simulink model "AeroCoeffsNew"  (R2020b)
settings: Solver=VariableStepAuto  StartTime=0.0  StopTime=50  FixedStep=0.1  RelTol=1e-3
values from neighbouring files (symbols this model uses):
  A_2 = [0  0  0; 0  0  0; 0  0  0]    [Angular_gust.mat]    (also in Linear_gust.mat; Real_Values.m = zeros(3); Trial_Script.m = zeros(3); TryingNewAeroCoeffs.m = zeros(3))
  A_kal = [0 0 0 0 0 0 0 0 0 0 0 0 ... (36 elements, 6x6)]    [Angular_gust.mat]    (also in Linear_gust.mat; Real_Values.m = [0 0 0 1 0 0; Trial_Script.m = [0 0 0 1 0 0; TryingNewAeroCoeffs.m = [0 0 0 1 0 0)
  B_2 = [0.0024294842205  2.57653534931e-06  6.44659625064e-05; 0  -0.000916808772026  -2.10833406567e-07; 0  0  -0.000799328564006]    [Angular_gust.mat]    (also in Linear_gust.mat; Real_Values.m = I_inv; Trial_Script.m = I_inv; TryingNewAeroCoeffs.m = I_inv)
  B_kal = [0 0 0 0 0 0 0 0 0 0 0 0 ... (36 elements, 6x6)]    [Angular_gust.mat]    (also in Linear_gust.mat; Real_Values.m = [0 0 0 0 0 0; Trial_Script.m = [0 0 0 0 0 0; TryingNewAeroCoeffs.m = [0 0 0 0 0 0)
  C_2 = [1  0  0; 0  1  0; 0  0  1]    [Angular_gust.mat]    (also in Linear_gust.mat; Real_Values.m = eye(3); Trial_Script.m = eye(3); TryingNewAeroCoeffs.m = eye(3))
  C_kal = [1 0 0 0 0 0 0 1 0 0 0 0 ... (36 elements, 6x6)]    [Angular_gust.mat]    (also in Linear_gust.mat; Real_Values.m = eye(6); Trial_Script.m = eye(6); TryingNewAeroCoeffs.m = eye(6))
  D_2 = [0  0  0; 0  0  0; 0  0  0]    [Angular_gust.mat]    (also in Linear_gust.mat; Real_Values.m = zeros(3); Trial_Script.m = zeros(3); TryingNewAeroCoeffs.m = zeros(3))
  D_kal = [0 0 0 0 0 0 0 0 0 0 0 0 ... (36 elements, 6x6)]    [Angular_gust.mat]    (also in Linear_gust.mat; Real_Values.m = zeros(6); Trial_Script.m = zeros(6); TryingNewAeroCoeffs.m = zeros(6))
  delta_time = 0.0178961433409    [Angular_gust.mat]    (also in Linear_gust.mat; Real_Values.m = time/length(xdata); Trial_Script.m = time/length(xdata); TryingNewAeroCoeffs.m = time/length(xdata))
  Fb1_l = -2600    [Angular_gust.mat]    (also in Linear_gust.mat; Real_Values.m = -260; Trial_Script.m; TryingNewAeroCoeffs.m)
  Fb1_u = 2600    [Angular_gust.mat]    (also in Linear_gust.mat; Real_Values.m = 260; Trial_Script.m; TryingNewAeroCoeffs.m)
  Fb2_l = -2600    [Angular_gust.mat]    (also in Linear_gust.mat; Real_Values.m = -260; Trial_Script.m; TryingNewAeroCoeffs.m)
  Fb2_u = 2600    [Angular_gust.mat]    (also in Linear_gust.mat; Real_Values.m = 260; Trial_Script.m; TryingNewAeroCoeffs.m)
  Fb3_l = -3200    [Angular_gust.mat]    (also in Linear_gust.mat; Real_Values.m = -320; Trial_Script.m; TryingNewAeroCoeffs.m)
  Fb3_u = 3200    [Angular_gust.mat]    (also in Linear_gust.mat; Real_Values.m = 320; Trial_Script.m; TryingNewAeroCoeffs.m)
  Fb4_l = -3200    [Angular_gust.mat]    (also in Linear_gust.mat; Real_Values.m = -320; Trial_Script.m; TryingNewAeroCoeffs.m)
  Fb4_u = 3200    [Angular_gust.mat]    (also in Linear_gust.mat; Real_Values.m = 320; Trial_Script.m; TryingNewAeroCoeffs.m)
  Fc1_l = -300    [Angular_gust.mat]    (also in Linear_gust.mat; Real_Values.m = -100; Trial_Script.m = -3000; TryingNewAeroCoeffs.m)
  Fc1_u = 300    [Angular_gust.mat]    (also in Linear_gust.mat; Real_Values.m = 100; Trial_Script.m = 3000; TryingNewAeroCoeffs.m)
  Fc2_l = -300    [Angular_gust.mat]    (also in Linear_gust.mat; Real_Values.m = -100; Trial_Script.m = -3000; TryingNewAeroCoeffs.m)
  Fc2_u = 300    [Angular_gust.mat]    (also in Linear_gust.mat; Real_Values.m = 100; Trial_Script.m = 3000; TryingNewAeroCoeffs.m)
  Fc3_l = -300    [Angular_gust.mat]    (also in Linear_gust.mat; Real_Values.m = -100; Trial_Script.m = -3000; TryingNewAeroCoeffs.m)
  Fc3_u = 300    [Angular_gust.mat]    (also in Linear_gust.mat; Real_Values.m = 100; Trial_Script.m = 3000; TryingNewAeroCoeffs.m)
  fprop = 1000    [Angular_gust.mat]    (also in Linear_gust.mat; TryingNewAeroCoeffs.m)
  Ft1_l = -5600    [Angular_gust.mat]    (also in Linear_gust.mat; Real_Values.m = -560; Trial_Script.m; TryingNewAeroCoeffs.m)
  Ft1_u = 5600    [Angular_gust.mat]    (also in Linear_gust.mat; Real_Values.m = 560; Trial_Script.m; TryingNewAeroCoeffs.m)
  Ft2_l = -5600    [Angular_gust.mat]    (also in Linear_gust.mat; Real_Values.m = -560; Trial_Script.m; TryingNewAeroCoeffs.m)
  Ft2_u = 5600    [Angular_gust.mat]    (also in Linear_gust.mat; Real_Values.m = 560; Trial_Script.m; TryingNewAeroCoeffs.m)
  Ft3_l = -3200    [Angular_gust.mat]    (also in Linear_gust.mat; Real_Values.m = -320; Trial_Script.m; TryingNewAeroCoeffs.m)
  Ft3_u = 3200    [Angular_gust.mat]    (also in Linear_gust.mat; Real_Values.m = 320; Trial_Script.m; TryingNewAeroCoeffs.m)
  Ft4_l = -3200    [Angular_gust.mat]    (also in Linear_gust.mat; Real_Values.m = -320; Trial_Script.m; TryingNewAeroCoeffs.m)
  Ft4_u = 3200    [Angular_gust.mat]    (also in Linear_gust.mat; Real_Values.m = 320; Trial_Script.m; TryingNewAeroCoeffs.m)
  g = 9.81    [Angular_gust.mat]    (also in Linear_gust.mat; Real_Values.m; Trial_Script.m; TryingNewAeroCoeffs.m)
  m = 941.102    [Angular_gust.mat]    (also in Linear_gust.mat; Real_Values.m; Trial_Script.m = 645; TryingNewAeroCoeffs.m)
  r_0 = [0 0 0]    [Angular_gust.mat]    (also in Linear_gust.mat; Real_Values.m = [0;0;0]; Trial_Script.m = [0;0;0]; TryingNewAeroCoeffs.m = [0;0;0])
  r_cgCatia = [0.0401998 0.00180957 -0.293434]    [Angular_gust.mat]    (also in Linear_gust.mat; Real_Values.m = TcgCatia*r_cgCatia; Trial_Script.m = [2; 0; 0]; TryingNewAeroCoeffs.m = TcgCatia*r_cgCatia)
  r_trajectory = [0 0 0]    [Angular_gust.mat]    (also in Linear_gust.mat; Real_Values.m = [0;0;0]; Trial_Script.m = [0;0;0]; TryingNewAeroCoeffs.m = [0;0;0])
  rho = 1.225    [Angular_gust.mat]    (also in Linear_gust.mat; Real_Values.m; Trial_Script.m; TryingNewAeroCoeffs.m)
  T = 10.5    [Angular_gust.mat]    (also in Linear_gust.mat; Real_Values.m; Trial_Script.m; TryingNewAeroCoeffs.m)
  t_finalgust = 17.9140394843    [Angular_gust.mat]    (also in Linear_gust.mat; Real_Values.m = time; TryingNewAeroCoeffs.m = time)
  TcgCatia = [1  0  0; 0  -1  0; 0  0  -1]    [Angular_gust.mat]    (also in Linear_gust.mat; Real_Values.m = [1 0 0; Trial_Script.m = [1 0 0; TryingNewAeroCoeffs.m = [1 0 0)
  time = 17.9140394843    [Angular_gust.mat]    (also in Linear_gust.mat; Real_Values.m = rdiff_abs/V0_shard; Trial_Script.m = abs(rdiff_shard(2)/V0_shard(2)); TryingNewAeroCoeffs.m = rdiff_abs/V0_shard)
  time_delay = 0.01    [Angular_gust.mat]    (also in Linear_gust.mat; Real_Values.m = 0.1; Trial_Script.m = 0.1; TryingNewAeroCoeffs.m)
  Tzy_Shard = [6.12323399574e-17  1  1.22464679915e-16; 1  -6.12323399574e-17  -7.49879891331e-33; 0  1.22464679915e-16  -1]    [Angular_gust.mat]    (also in Linear_gust.mat; Real_Values.m = [cos(pi/2) -sin(pi/2) 0; sin(pi/2) cos(pi/2) 0; 0 0 1]*[1 0 ; Trial_Script.m = [cos(pi/2) -sin(pi/2) 0; sin(pi/2) cos(pi/2) 0; 0 0 1]*[1 0 ; TryingNewAeroCoeffs.m = [cos(pi/2) -sin(pi/2) 0; sin(pi/2) cos(pi/2) 0; 0 0 1]*[1 0 )
  u0_final = 23.9559    [Angular_gust.mat]    (also in Linear_gust.mat; Real_Values.m = u_0(length(u_0)); TryingNewAeroCoeffs.m = u_0(length(u_0)))
  u1_final = -0.480858    [Angular_gust.mat]    (also in Linear_gust.mat; Real_Values.m = u_1(length(u_1)); TryingNewAeroCoeffs.m = u_1(length(u_1)))
  u2_final = -0.725589    [Angular_gust.mat]    (also in Linear_gust.mat; Real_Values.m = u_2(length(u_2)); TryingNewAeroCoeffs.m = u_2(length(u_2)))
  u_0 = [24.7775 24.7775 24.7775 24.7775 24.7775 24.7775 24.7775 24.7775 24.7775 24.7775 24.7775 24.7775 ... (1001 elements, 1001x1)]    [Angular_gust.mat]    (also in Linear_gust.mat; Real_Values.m = a(1:d_shard,1); Trial_Script.m = a(1:d_shard,1); TryingNewAeroCoeffs.m = a(1:d_shard,1))
  u_1 = [0.712897 0.712897 0.712897 0.712897 0.712897 0.712897 0.712897 0.712897 0.712897 0.712897 0.712897 0.712897 ... (1001 elements, 1001x1)]    [Angular_gust.mat]    (also in Linear_gust.mat; Real_Values.m = a(1:d_shard,2); Trial_Script.m = a(1:d_shard,2); TryingNewAeroCoeffs.m = a(1:d_shard,2))
  u_2 = [-0.504815 -0.504815 -0.504815 -0.504815 -0.504815 -0.504815 -0.504815 -0.504815 -0.504815 -0.504815 -0.504815 -0.504815 ... (1001 elements, 1001x1)]    [Angular_gust.mat]    (also in Linear_gust.mat; Real_Values.m = a(1:d_shard,3); Trial_Script.m = a(1:d_shard,3); TryingNewAeroCoeffs.m = a(1:d_shard,3))
  v_0 = [0 0 0]    [Angular_gust.mat]    (also in Linear_gust.mat; Real_Values.m = [0;0;0]; Trial_Script.m = [0;0;0]; TryingNewAeroCoeffs.m = [0;0;0])
  ZI_Cx = [4.10002314469 4.10486511138 4.10970707807 4.11454904475 4.11939101144 4.12423297813 4.12907494481 4.1339169115 4.13875887819 4.14360084487 4.14844281156 4.15328477825 ... (65341 elements, 361x181)]    [Angular_gust.mat]    (also in Linear_gust.mat; Real_Values.m = model_Cx(XI_Cx, YI_Cx); Trial_Script.m = model_Cx(XI_Cx, YI_Cx); TryingNewAeroCoeffs.m = model_Cx(XI_Cx, YI_Cx))
  ZI_Cy = [5.10662222372 5.15407485934 5.20152749496 5.24898013059 5.29643276621 5.34388540184 5.39133803746 5.43879067308 5.48624330871 5.53369594433 5.58114857996 5.62860121558 ... (65341 elements, 361x181)]    [Angular_gust.mat]    (also in Linear_gust.mat; Real_Values.m = model_Cy(XI_Cy, YI_Cy); Trial_Script.m = model_Cy(XI_Cy, YI_Cy); TryingNewAeroCoeffs.m = model_Cy(XI_Cy, YI_Cy))
  ZI_Cz = [-10.5947720774 -10.6317912004 -10.6688103235 -10.7058294465 -10.7428485695 -10.7798676926 -10.8168868156 -10.8539059387 -10.8909250617 -10.9279441847 -10.9649633078 -11.0019824308 ... (65341 elements, 361x181)]    [Angular_gust.mat]    (also in Linear_gust.mat; Real_Values.m = model_Cz(XI_Cz, YI_Cz); Trial_Script.m = model_Cz(XI_Cz, YI_Cz); TryingNewAeroCoeffs.m = model_Cz(XI_Cz, YI_Cz))
  ZI_p = [6.05111971338 6.06712776392 6.08313581446 6.099143865 6.11515191553 6.13115996607 6.14716801661 6.16317606715 6.17918411769 6.19519216823 6.21120021877 6.22720826931 ... (65341 elements, 361x181)]    [Angular_gust.mat]    (also in Linear_gust.mat; Real_Values.m = model_p(XI_p, YI_p); Trial_Script.m = model_p(XI_p, YI_p); TryingNewAeroCoeffs.m = model_p(XI_p, YI_p))
  ZI_q = [0.071083987219 0.054175962948 0.0372679386771 0.0203599144061 0.00345189013513 -0.0134561341358 -0.0303641584068 -0.0472721826778 -0.0641802069487 -0.0810882312197 -0.0979962554907 -0.114904279762 ... (65341 elements, 361x181)]    [Angular_gust.mat]    (also in Linear_gust.mat; Real_Values.m = model_q(XI_q, YI_q); Trial_Script.m = model_q(XI_q, YI_q); TryingNewAeroCoeffs.m = model_q(XI_q, YI_q))
  ZI_r = [-1.8762921931 -1.88364224017 -1.89099228723 -1.8983423343 -1.90569238136 -1.91304242842 -1.92039247549 -1.92774252255 -1.93509256961 -1.94244261668 -1.94979266374 -1.95714271081 ... (65341 elements, 361x181)]    [Angular_gust.mat]    (also in Linear_gust.mat; Real_Values.m = model_r(XI_r, YI_r); Trial_Script.m = model_r(XI_r, YI_r); TryingNewAeroCoeffs.m = model_r(XI_r, YI_r))
undefined symbols (not defined in the file or in its folder): Continuous, Time
libraries: dspsigops x11, simulink x9, fuzblock x3, pid_lib x3, sharedutil x1, mpclib x1, cstblocks x1, dspmathops x1, ctrlSharedLib x1
(part 1 of 2)
settings Model: Creator=Jonathan van Zyl  LastModifiedBy=Jonathan van Zyl

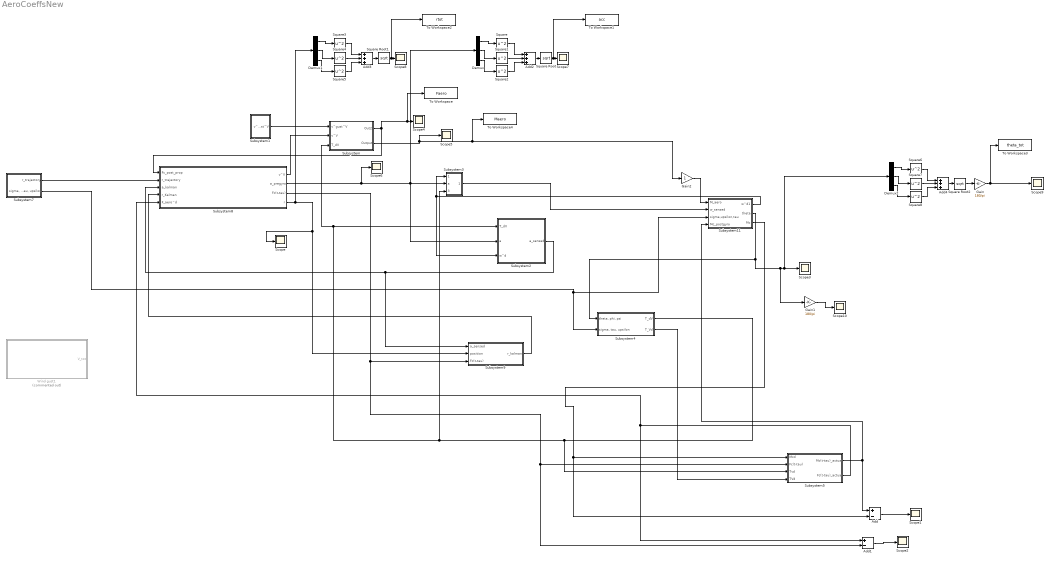
== system AeroCoeffsNew ==
  Add : Sum  Inputs=+-
  Add1 : Sum  Inputs=+-
  Add2 : Sum  Inputs=+++
  Add3 : Sum  Inputs=+++
  Add4 : Sum  Inputs=+++
  Demux : Demux  Outputs=3
  Demux1 : Demux  Outputs=3
  Demux2 : Demux  Outputs=3
  Gain : Gain  Gain=180/pi
  Gain1 : Gain  Gain=180/pi
  Gain2 : Gain
  Scope{,1..10} (11 alike) : Scope
  Square{,1..8} (9 alike) : Math  Operator=square  SaturateOnIntegerOverflow=on
  Square Root : Sqrt  SaturateOnIntegerOverflow=on
  Square Root1 : Sqrt  SaturateOnIntegerOverflow=on
  Square Root2 : Sqrt  SaturateOnIntegerOverflow=on
  Subsystem : Subsystem
  Subsystem1 : Subsystem
  Subsystem11 : Subsystem
  Subsystem2 : Subsystem
  Subsystem3 : Subsystem
  Subsystem4 : Subsystem
  Subsystem5 : Subsystem
  Subsystem7 : Subsystem
  Subsystem8 : Subsystem
  Subsystem9 : Subsystem
  To Workspace : ToWorkspace  VariableName=Faero  SaveFormat=Timeseries  SampleTime=-1
  To Workspace1 : ToWorkspace  VariableName=acc  SaveFormat=Timeseries  SampleTime=-1
  To Workspace2 : ToWorkspace  VariableName=rtot  SaveFormat=Timeseries  SampleTime=-1
  To Workspace3 : ToWorkspace  VariableName=theta_tot  SaveFormat=Timeseries  SampleTime=-1
  To Workspace4 : ToWorkspace  VariableName=Maero  SaveFormat=Timeseries  SampleTime=-1
  Wind gust1 : Subsystem  Commented=on
  wires:
  Subsystem2/1(a_sensed) -> Subsystem8/3(a_kalman), Subsystem9/1(a_sensed)
  Subsystem/2(Output) -> Scope5/1, Gain2/1, To Workspace4/1
  Subsystem/1(Out2) -> To Workspace/1, Scope4/1, Subsystem8/1(Fc_post_prop)
  Subsystem1/1(v^gust^V) -> Subsystem/1(v^gust^V)
  Subsystem4/1(T_dV) -> Subsystem5/3(Tvd), Subsystem/3(T_dV), Subsystem2/1(T_dV), Subsystem3/3(T_dV)
  Subsystem4/2(T_Vd) -> Subsystem5/4(TVd)
  Subsystem7/2("sigma, tau, upsilon") -> Subsystem11/3(sigma,upsilon,tau), Subsystem4/2("sigma, tau, upsilon")
  Subsystem8/3(Fc(t-tau)) -> Add1/2, Subsystem5/2(Fc(t-tau)), Subsystem9/3(Fc(t-tau))
  Subsystem7/1(r_trajectory) -> Subsystem8/2(r_trajectory)
  Subsystem5/2(Fc(t-tau)_actual) -> Add1/1, Subsystem8/5(F_aero^d)
  Subsystem8/1(v^V) -> Subsystem/2(v^V)
  Subsystem11/1(w^d1) -> Subsystem2/3(w^d), Subsystem3/1(w^d)
  Subsystem3/1(w^d1) -> Subsystem11/2(w_sensed)
  Subsystem5/1(Mc(t-tau)_actual) -> Subsystem11/4(Mc_postgyro), Add/1
  Subsystem11/3(Mc) -> Add/2, Subsystem5/1(Mcd)
  Subsystem9/1(r_kalman) -> Subsystem8/4(r_Kalman)
  Add/1 -> Scope1/1
  Add1/1 -> Scope2/1
  Demux/2 -> Square1/1
  Subsystem8/2(a_pregyro) -> Scope6/1, Demux/1, Subsystem3/2(a), Subsystem2/2(a)
  Demux/1 -> Square/1
  Demux/3 -> Square2/1
  Square Root/1 -> To Workspace1/1, Scope7/1
  Add2/1 -> Square Root/1
  Square2/1 -> Add2/3
  Square/1 -> Add2/1
  Square1/1 -> Add2/2
  Subsystem8/4(r) -> Demux1/1, Scope/1, Subsystem9/2(position)
  Demux1/2 -> Square4/1
  Demux1/1 -> Square3/1
  Add3/1 -> Square Root1/1
  Square4/1 -> Add3/2
  Square Root1/1 -> To Workspace2/1, Scope8/1
  Square3/1 -> Add3/1
  Demux1/3 -> Square5/1
  Square5/1 -> Add3/3
  Subsystem11/2(theta) -> Gain1/1, Demux2/1, Scope3/1, Subsystem4/1("theta, phi, psi")
  Demux2/2 -> Square7/1
  Demux2/1 -> Square6/1
  Add4/1 -> Square Root2/1
  Square7/1 -> Add4/2
  Gain/1 -> To Workspace3/1, Scope9/1
  Square6/1 -> Add4/1
  Demux2/3 -> Square8/1
  Square8/1 -> Add4/3
  Square Root2/1 -> Gain/1
  Gain1/1 -> Scope10/1
  Gain2/1 -> Subsystem11/1(M_aero)

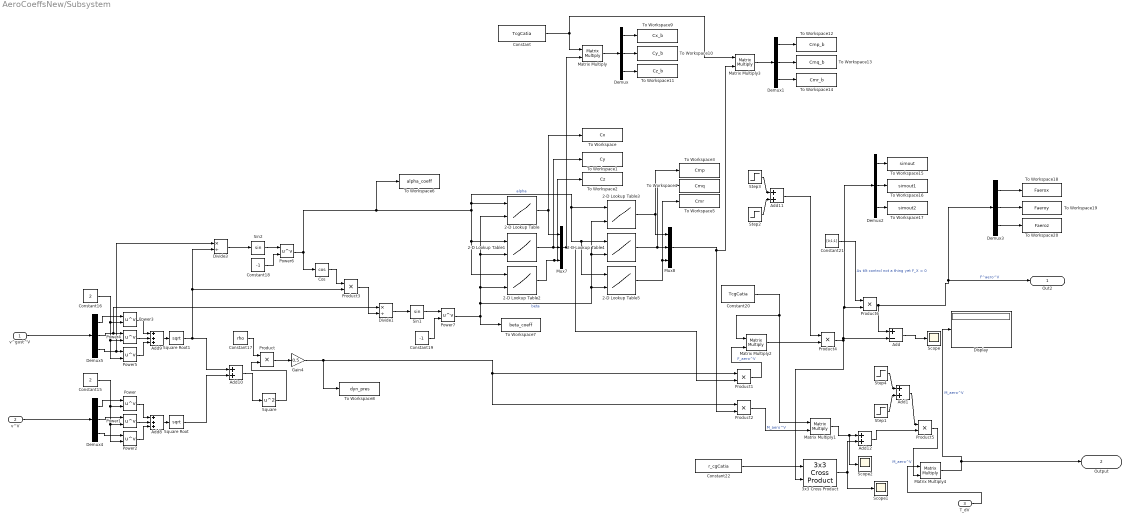
== system AeroCoeffsNew/Subsystem ==
  v^gust^V : Inport
  v^V : Inport  Port=2
  T_dV : Inport  Port=3
  2-D Lookup Table : Lookup_n-D  BreakpointsForDimension1=[-180:1:180]  BreakpointsForDimension2=[-90:1:90]  Table=ZI_Cx  InternalRulePriority=Speed  RndMeth=Simplest  InputSameDT=on
      settings: InputPortMap=u0,u1
  2-D Lookup Table1 : Lookup_n-D  BreakpointsForDimension1=[-180:1:180]  BreakpointsForDimension2=[-90:1:90]  Table=ZI_Cy  InternalRulePriority=Speed  RndMeth=Simplest  InputSameDT=on
      settings: InputPortMap=u0,u1
  2-D Lookup Table2 : Lookup_n-D  BreakpointsForDimension1=[-180:1:180]  BreakpointsForDimension2=[-90:1:90]  Table=ZI_Cz  InternalRulePriority=Speed  RndMeth=Simplest  InputSameDT=on
      settings: InputPortMap=u0,u1
  2-D Lookup Table3 : Lookup_n-D  BreakpointsForDimension1=[-180:1:180]  BreakpointsForDimension2=[-90:1:90]  Table=ZI_p  InternalRulePriority=Speed  RndMeth=Simplest  InputSameDT=on
      settings: InputPortMap=u0,u1
  2-D Lookup Table4 : Lookup_n-D  BreakpointsForDimension1=[-180:1:180]  BreakpointsForDimension2=[-90:1:90]  Table=ZI_q  InternalRulePriority=Speed  RndMeth=Simplest  InputSameDT=on
      settings: InputPortMap=u0,u1
  2-D Lookup Table5 : Lookup_n-D  BreakpointsForDimension1=[-180:1:180]  BreakpointsForDimension2=[-90:1:90]  Table=ZI_r  InternalRulePriority=Speed  RndMeth=Simplest  InputSameDT=on
      settings: InputPortMap=u0,u1
  3x3 Cross Product : sharedutil/3x3 Cross Product  aMode=aMode
      settings: SourceProductBaseCode=AE,PW,MT,UV,VE,VP
  Add : Sum  Inputs=+-
  Add{1,10..12} (4 alike) : Sum
  Add8 : Sum  Inputs=+++
  Add9 : Sum  Inputs=+++
  Constant : Constant  Value=TcgCatia
  Constant15 : Constant  Value=2
  Constant16 : Constant  Value=2
  Constant17 : Constant  Value=rho
  Constant18 : Constant  Value=-1
  Constant19 : Constant  Value=-1
  Constant20 : Constant  Value=TcgCatia
  Constant21 : Constant  Value=[0;1;1]
  Constant22 : Constant  Value=r_cgCatia
  Cos : Trigonometry  Operator=cos
  Demux{,1..5} (6 alike) : Demux  Outputs=3
  Display : Display
  Divide1 : Product  Inputs=*/
  Divide3 : Product  Inputs=*/
  Gain4 : Gain  Gain=0.5
  Matrix Multiply{,1..4} (5 alike) : Product  Multiplication=Matrix(*)
  Mux7 : Mux  Inputs=3
  Mux8 : Mux  Inputs=3
  Power{,1..7} (8 alike) : Math  Operator=pow  SaturateOnIntegerOverflow=on
  Product{,1..6} (7 alike) : Product
  Scope : Scope
  Scope1 : Scope
  Scope2 : Scope
  Sin1 : Trigonometry
  Sin2 : Trigonometry
  Square : Math  Operator=square  SaturateOnIntegerOverflow=on
  Square Root : Sqrt  SaturateOnIntegerOverflow=on
  Square Root1 : Sqrt  SaturateOnIntegerOverflow=on
  Step1 : Step  Time=0  SampleTime=0
  Step2 : Step  Time=0  SampleTime=0
  Step3 : Step  Time=time  After=-1  SampleTime=0
  Step4 : Step  Time=time  After=-1  SampleTime=0
  To Workspace : ToWorkspace  VariableName=Cx  SaveFormat=Timeseries  SampleTime=-1
  To Workspace1 : ToWorkspace  VariableName=Cy  SaveFormat=Timeseries  SampleTime=-1
  To Workspace10 : ToWorkspace  VariableName=Cy_b  SaveFormat=Timeseries  SampleTime=-1
  To Workspace11 : ToWorkspace  VariableName=Cz_b  SaveFormat=Timeseries  SampleTime=-1
  To Workspace12 : ToWorkspace  VariableName=Cmp_b  SaveFormat=Timeseries  SampleTime=-1
  To Workspace13 : ToWorkspace  VariableName=Cmq_b  SaveFormat=Timeseries  SampleTime=-1
  To Workspace14 : ToWorkspace  VariableName=Cmr_b  SaveFormat=Timeseries  SampleTime=-1
  To Workspace15 : ToWorkspace  VariableName=simout  SaveFormat=Timeseries  SampleTime=-1
  To Workspace16 : ToWorkspace  VariableName=simout1  SaveFormat=Timeseries  SampleTime=-1
  To Workspace17 : ToWorkspace  VariableName=simout2  SaveFormat=Timeseries  SampleTime=-1
  To Workspace18 : ToWorkspace  VariableName=Faerox  SaveFormat=Timeseries  SampleTime=-1
  To Workspace19 : ToWorkspace  VariableName=Faeroy  SaveFormat=Timeseries  SampleTime=-1
  To Workspace2 : ToWorkspace  VariableName=Cz  SaveFormat=Timeseries  SampleTime=-1
  To Workspace20 : ToWorkspace  VariableName=Faeroz  SaveFormat=Timeseries  SampleTime=-1
  To Workspace3 : ToWorkspace  VariableName=Cmp  SaveFormat=Timeseries  SampleTime=-1
  To Workspace4 : ToWorkspace  VariableName=Cmq  SaveFormat=Timeseries  SampleTime=-1
  To Workspace5 : ToWorkspace  VariableName=Cmr  SaveFormat=Timeseries  SampleTime=-1
  To Workspace6 : ToWorkspace  VariableName=alpha_coeff  SaveFormat=Timeseries  SampleTime=-1
  To Workspace7 : ToWorkspace  VariableName=beta_coeff  SaveFormat=Timeseries  SampleTime=-1
  To Workspace8 : ToWorkspace  VariableName=dyn_pres  SaveFormat=Timeseries  SampleTime=-1
  To Workspace9 : ToWorkspace  VariableName=Cx_b  SaveFormat=Timeseries  SampleTime=-1
  Out2 : Outport
  Output : Outport  Port=2
  wires:
  Demux5/1 -> Power3/1
  Constant21/1 -> Product6/1  "As tilt control not a thing yet F_X = 0"
  2-D Lookup Table3/1 -> To Workspace3/1, Mux8/1
  Constant17/1 -> Product/1
  Power5/1 -> Add9/3
  Product4/1 -> Demux2/1, Product6/2, Add/2, 3x3 Cross Product/2
  Power7/1 -> 2-D Lookup Table/2, 2-D Lookup Table1/2, 2-D Lookup Table2/2, 2-D Lookup Table3/2, 2-D Lookup Table4/2, 2-D Lookup Table5/2, To Workspace7/1  "beta"
  2-D Lookup Table2/1 -> To Workspace2/1, Mux7/3
  Power3/1 -> Add9/1
  Constant15/1 -> Power2/2, Power1/2, Power/2
  Sin1/1 -> Power7/1
  Square/1 -> Product/2
  Demux4/2 -> Power1/1
  Gain4/1 -> To Workspace8/1, Product2/1, Product1/1
  Square Root1/1 -> Product3/2, Divide3/2, Add10/1
  Product1/1 -> Matrix Multiply2/2  "F_aero^V"
  2-D Lookup Table1/1 -> To Workspace1/1, Mux7/2
  Add8/1 -> Square Root/1
  Cos/1 -> Product3/1
  3x3 Cross Product/1 -> Add12/2, Scope1/1
  Power2/1 -> Add8/3
  Add9/1 -> Square Root1/1
  Divide3/1 -> Sin2/1
  Mux7/1 -> Matrix Multiply/2, Product1/2
  Demux5/2 -> Divide1/1, Power4/1
  Product3/1 -> Divide1/2
  Constant22/1 -> 3x3 Cross Product/1
  Product2/1 -> Matrix Multiply1/2  "M_aero^V"
  Demux4/3 -> Power2/1
  Square Root/1 -> Add10/2
  Constant16/1 -> Power5/2, Power4/2, Power3/2
  2-D Lookup Table5/1 -> To Workspace5/1, Mux8/3
  v^gust^V/1 -> Demux5/1
  Divide1/1 -> Sin1/1
  Power1/1 -> Add8/2
  Constant20/1 -> Matrix Multiply1/1, Matrix Multiply2/1
  Power4/1 -> Add9/2
  Power/1 -> Add8/1
  2-D Lookup Table4/1 -> To Workspace4/1, Mux8/2
  Matrix Multiply1/1 -> Scope2/1, Add12/1
  Mux8/1 -> Matrix Multiply3/2, Product2/2
  Constant18/1 -> Power6/2
  Demux4/1 -> Power/1
  Product6/1 -> Add/1, Out2/1, Demux3/1  "F^aero^V"
  Demux5/3 -> Divide3/1, Power5/1
  Product/1 -> Gain4/1
  Power6/1 -> Cos/1, To Workspace6/1, 2-D Lookup Table/1, 2-D Lookup Table5/1, 2-D Lookup Table4/1, 2-D Lookup Table3/1, 2-D Lookup Table2/1, 2-D Lookup Table1/1  "alpha"
  Sin2/1 -> Power6/1
  Constant19/1 -> Power7/2
  2-D Lookup Table/1 -> Mux7/1, To Workspace/1
  Add10/1 -> Square/1
  Matrix Multiply4/1 -> Display/1, Output/1  "M_aero^V"
  T_dV/1 -> Matrix Multiply4/1
  v^V/1 -> Demux4/1
  Add/1 -> Scope/1
  Constant/1 -> Matrix Multiply3/1, Matrix Multiply/1
  Matrix Multiply/1 -> Demux/1
  Demux/1 -> To Workspace9/1
  Demux/2 -> To Workspace10/1
  Demux/3 -> To Workspace11/1
  Matrix Multiply3/1 -> Demux1/1
  Demux1/1 -> To Workspace12/1
  Demux1/2 -> To Workspace13/1
  Demux1/3 -> To Workspace14/1
  Demux2/1 -> To Workspace15/1
  Demux2/2 -> To Workspace16/1
  Demux2/3 -> To Workspace17/1
  Demux3/1 -> To Workspace18/1
  Demux3/2 -> To Workspace19/1
  Demux3/3 -> To Workspace20/1
  Step3/1 -> Add11/1
  Add11/1 -> Product4/1
  Step2/1 -> Add11/2
  Matrix Multiply2/1 -> Product4/2
  Add1/1 -> Product5/1
  Step1/1 -> Add1/2
  Step4/1 -> Add1/1
  Product5/1 -> Matrix Multiply4/2  "M_aero^V"
  Add12/1 -> Product5/2

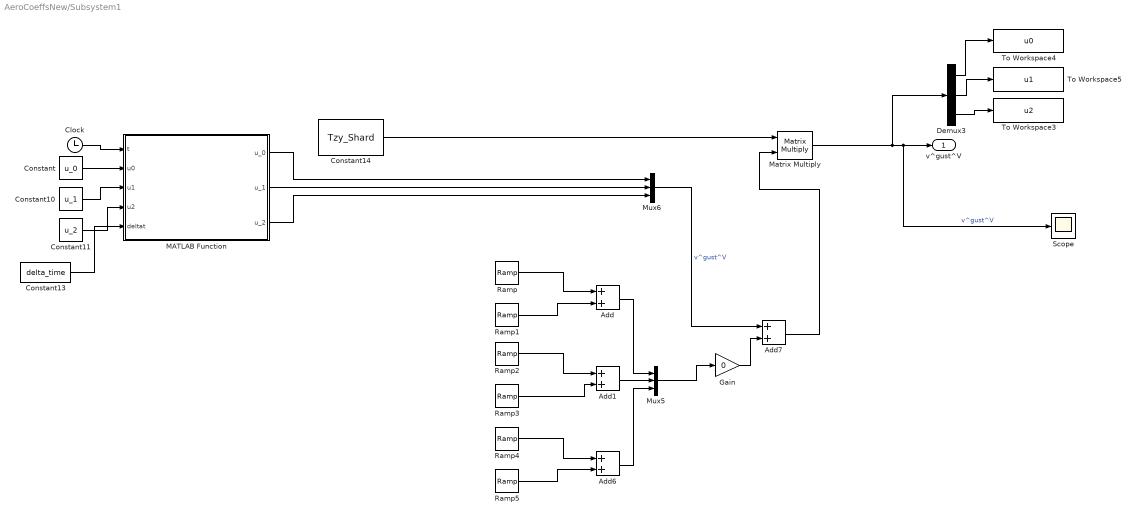
== system AeroCoeffsNew/Subsystem1 ==
  Add{,1,6..7} (4 alike) : Sum
  Clock : Clock
  Constant : Constant  Value=u_0
  Constant10 : Constant  Value=u_1
  Constant11 : Constant  Value=u_2
  Constant13 : Constant  Value=delta_time
  Constant14 : Constant  Value=Tzy_Shard
  Demux3 : Demux  Outputs=3
  Gain : Gain  Gain=0
  MATLAB Function : MATLAB Function  TreatAsAtomicUnit=on
  Matrix Multiply : Product  Multiplication=Matrix(*)
  Mux5 : Mux  Inputs=3
  Mux6 : Mux  Inputs=3
  Ramp : simulink/Sources/Ramp  slope=-1  start=t_finalgust  InitialOutput=0
  Ramp1 : simulink/Sources/Ramp  slope=1  start=t_finalgust + u0_final  InitialOutput=0
  Ramp2 : simulink/Sources/Ramp  slope=-1  start=t_finalgust  InitialOutput=0
  Ramp3 : simulink/Sources/Ramp  slope=1  start=t_finalgust + u1_final  InitialOutput=0
  Ramp4 : simulink/Sources/Ramp  slope=-1  start=t_finalgust  InitialOutput=0
  Ramp5 : simulink/Sources/Ramp  slope=1  start=t_finalgust + u2_final  InitialOutput=0
  Scope : Scope
  To Workspace3 : ToWorkspace  VariableName=u2  SaveFormat=Timeseries  SampleTime=-1
  To Workspace4 : ToWorkspace  VariableName=u0  SaveFormat=Timeseries  SampleTime=-1
  To Workspace5 : ToWorkspace  VariableName=u1  SaveFormat=Timeseries  SampleTime=-1
  v^gust^V : Outport
  wires:
  Add1/1 -> Mux5/2
  MATLAB Function/1(u_0) -> Mux6/1
  Add7/1 -> Matrix Multiply/2
  Constant13/1 -> MATLAB Function/5(deltat)
  Ramp4/1 -> Add6/1
  Ramp3/1 -> Add1/2
  Constant11/1 -> MATLAB Function/4(u2)
  Constant/1 -> MATLAB Function/2(u0)
  Ramp1/1 -> Add/2
  Mux5/1 -> Gain/1
  Constant14/1 -> Matrix Multiply/1
  MATLAB Function/2(u_1) -> Mux6/2
  Constant10/1 -> MATLAB Function/3(u1)
  Ramp/1 -> Add/1
  Matrix Multiply/1 -> Demux3/1, Scope/1, v^gust^V/1  "v^gust^V"
  Ramp5/1 -> Add6/2
  Add6/1 -> Mux5/3
  Clock/1 -> MATLAB Function/1(t)
  MATLAB Function/3(u_2) -> Mux6/3
  Add/1 -> Mux5/1
  Ramp2/1 -> Add1/1
  Mux6/1 -> Add7/1  "v^gust^V"
  Demux3/3 -> To Workspace3/1
  Demux3/2 -> To Workspace5/1
  Demux3/1 -> To Workspace4/1
  Gain/1 -> Add7/2

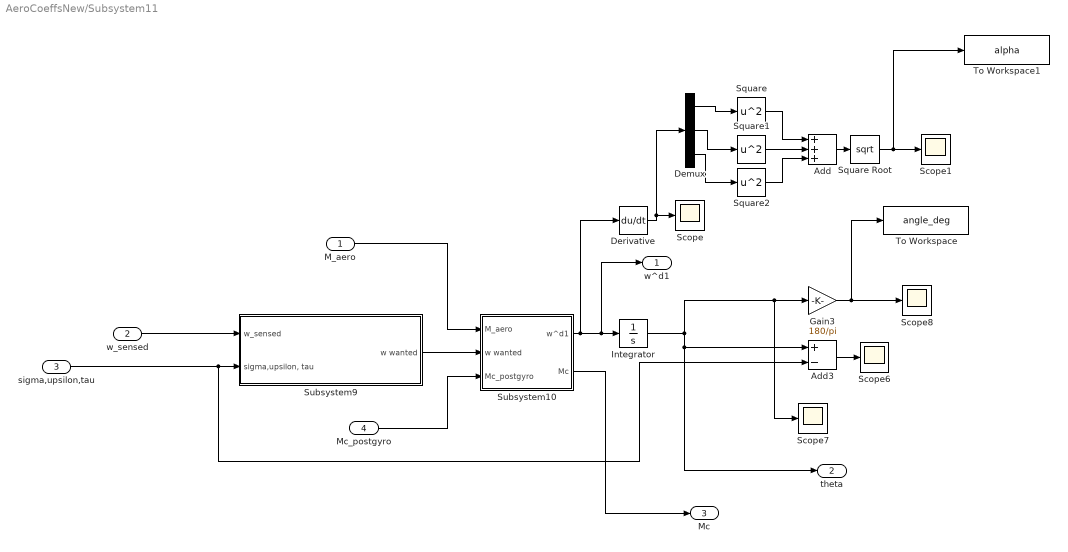
== system AeroCoeffsNew/Subsystem11 ==
  M_aero : Inport
  w_sensed : Inport  Port=2
  sigma,upsilon,tau : Inport  Port=3
  Mc_postgyro : Inport  Port=4
  Add : Sum  Inputs=+++
  Add3 : Sum  Inputs=+-
  Demux : Demux  Outputs=3
  Derivative : Derivative
  Gain3 : Gain  Gain=180/pi
  Integrator : Integrator
  Scope{,1,6..8} (5 alike) : Scope
  Square : Math  Operator=square  SaturateOnIntegerOverflow=on
  Square Root : Sqrt  SaturateOnIntegerOverflow=on
  Square1 : Math  Operator=square  SaturateOnIntegerOverflow=on
  Square2 : Math  Operator=square  SaturateOnIntegerOverflow=on
  Subsystem10 : Subsystem
  Subsystem9 : Subsystem
  To Workspace : ToWorkspace  VariableName=angle_deg  SaveFormat=Timeseries  SampleTime=-1
  To Workspace1 : ToWorkspace  VariableName=alpha  SaveFormat=Timeseries  SampleTime=-1
  w^d1 : Outport
  theta : Outport  Port=2
  Mc : Outport  Port=3
  wires:
  Gain3/1 -> To Workspace/1, Scope8/1
  M_aero/1 -> Subsystem10/1(M_aero)
  w_sensed/1 -> Subsystem9/1(w_sensed)
  Subsystem10/1(w^d1) -> Derivative/1, w^d1/1, Integrator/1
  sigma,upsilon,tau/1 -> Add3/2, Subsystem9/2("sigma,upsilon, tau")
  Integrator/1 -> theta/1, Add3/1, Gain3/1, Scope7/1
  Subsystem10/2(Mc) -> Mc/1
  Subsystem9/1(w wanted) -> Subsystem10/2(w wanted)
  Add3/1 -> Scope6/1
  Mc_postgyro/1 -> Subsystem10/3(Mc_postgyro)
  Derivative/1 -> Demux/1, Scope/1
  Demux/1 -> Square/1
  Demux/2 -> Square1/1
  Demux/3 -> Square2/1
  Square/1 -> Add/1
  Square1/1 -> Add/2
  Square2/1 -> Add/3
  Add/1 -> Square Root/1
  Square Root/1 -> To Workspace1/1, Scope1/1

== system AeroCoeffsNew/Subsystem2 ==
  T_dV : Inport
  a : Inport  Port=2
  w^d : Inport  Port=3
  Display1 : Display
  Display2 : Display
  MATLAB Function1 : MATLAB Function  Commented=on  TreatAsAtomicUnit=on
  Terminator5 : Terminator
  Terminator6 : Terminator
  Transpose1 : Math  Operator=transpose  SaturateOnIntegerOverflow=on
  Transpose2 : Math  Operator=transpose  SaturateOnIntegerOverflow=on
  Transpose3 : Math  Operator=transpose  SaturateOnIntegerOverflow=on
  a_sensed : Outport
  wires:
  a/1 -> Transpose1/1
  Transpose1/1 -> Display1/1, Transpose2/1, Display2/1  "a_sensed"
  Transpose3/1 -> Terminator5/1
  T_dV/1 -> Terminator6/1
  Transpose2/1 -> a_sensed/1  "a_sensed"
  w^d/1 -> Transpose3/1

== system AeroCoeffsNew/Subsystem3 ==
  w^d : Inport
  a : Inport  Port=2
  T_dV : Inport  Port=3
  Add : Sum  Inputs=+-
  Demux21 : Demux  Outputs=3
  Demux22 : Demux  Outputs=3
  MATLAB Function10 : MATLAB Function  TreatAsAtomicUnit=on
  Matrix Multiply4 : Product  Multiplication=Matrix(*)
  Mux14 : Mux  Inputs=3
  To Workspace : ToWorkspace  VariableName=gyro  SaveFormat=Timeseries  SampleTime=-1
  w^d1 : Outport
  wires:
  Demux21/3 -> MATLAB Function10/3(zvel)
  Demux22/1 -> MATLAB Function10/4(accx)
  Demux22/2 -> MATLAB Function10/5(accy)
  Demux22/3 -> MATLAB Function10/6(accz)
  MATLAB Function10/1(wx) -> Mux14/1
  Demux21/1 -> MATLAB Function10/1(xvel)
  MATLAB Function10/2(wy) -> Mux14/2
  Demux21/2 -> MATLAB Function10/2(yvel)
  MATLAB Function10/3(wz) -> Mux14/3
  Matrix Multiply4/1 -> Demux22/1
  Mux14/1 -> Add/2, w^d1/1  "w^d"
  T_dV/1 -> Matrix Multiply4/1
  a/1 -> Matrix Multiply4/2
  w^d/1 -> Add/1, Demux21/1
  Add/1 -> To Workspace/1

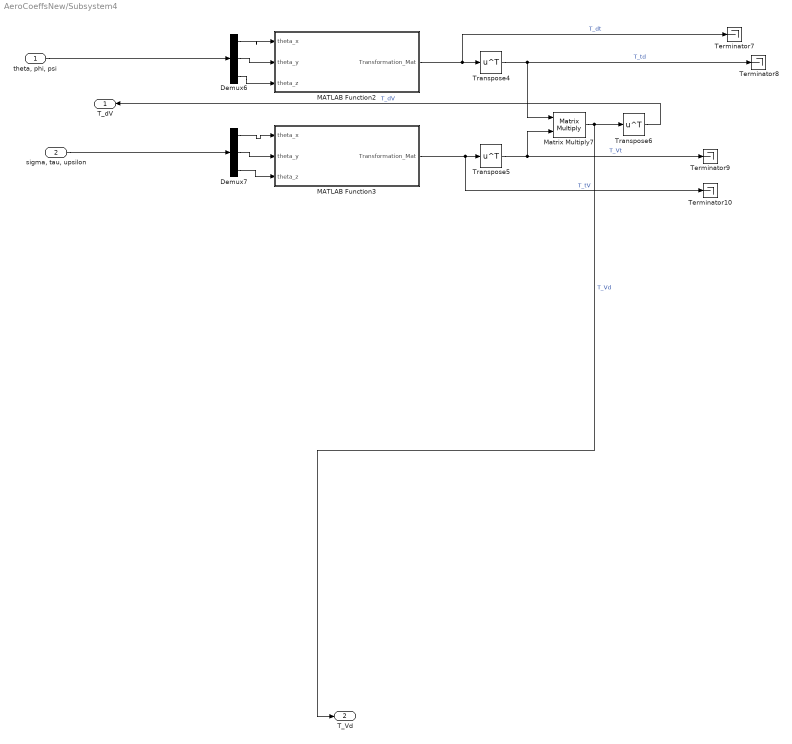
== system AeroCoeffsNew/Subsystem4 ==
  "theta, phi, psi" : Inport
  "sigma, tau, upsilon" : Inport  Port=2
  Demux6 : Demux  Outputs=3
  Demux7 : Demux  Outputs=3
  MATLAB Function2 : MATLAB Function  TreatAsAtomicUnit=on
  MATLAB Function3 : MATLAB Function  TreatAsAtomicUnit=on
  Matrix Multiply7 : Product  Multiplication=Matrix(*)
  Terminator{7..10} (4 alike) : Terminator
  Transpose4 : Math  Operator=transpose  SaturateOnIntegerOverflow=on
  Transpose5 : Math  Operator=transpose  SaturateOnIntegerOverflow=on
  Transpose6 : Math  Operator=transpose  SaturateOnIntegerOverflow=on
  T_dV : Outport
  T_Vd : Outport  Port=2
  wires:
  Matrix Multiply7/1 -> T_Vd/1, Transpose6/1  "T_Vd"
  Demux7/1 -> MATLAB Function3/1(theta_x)
  "theta, phi, psi"/1 -> Demux6/1
  Demux6/3 -> MATLAB Function2/3(theta_z)
  Demux7/3 -> MATLAB Function3/3(theta_z)
  "sigma, tau, upsilon"/1 -> Demux7/1
  Demux6/1 -> MATLAB Function2/1(theta_x)
  Transpose5/1 -> Terminator9/1, Matrix Multiply7/2  "T_Vt"
  MATLAB Function2/1(Transformation_Mat) -> Terminator7/1, Transpose4/1  "T_dt"
  Transpose4/1 -> Terminator8/1, Matrix Multiply7/1  "T_td"
  MATLAB Function3/1(Transformation_Mat) -> Terminator10/1, Transpose5/1  "T_tV"
  Demux6/2 -> MATLAB Function2/2(theta_y)
  Demux7/2 -> MATLAB Function3/2(theta_y)
  Transpose6/1 -> T_dV/1  "T_dV"

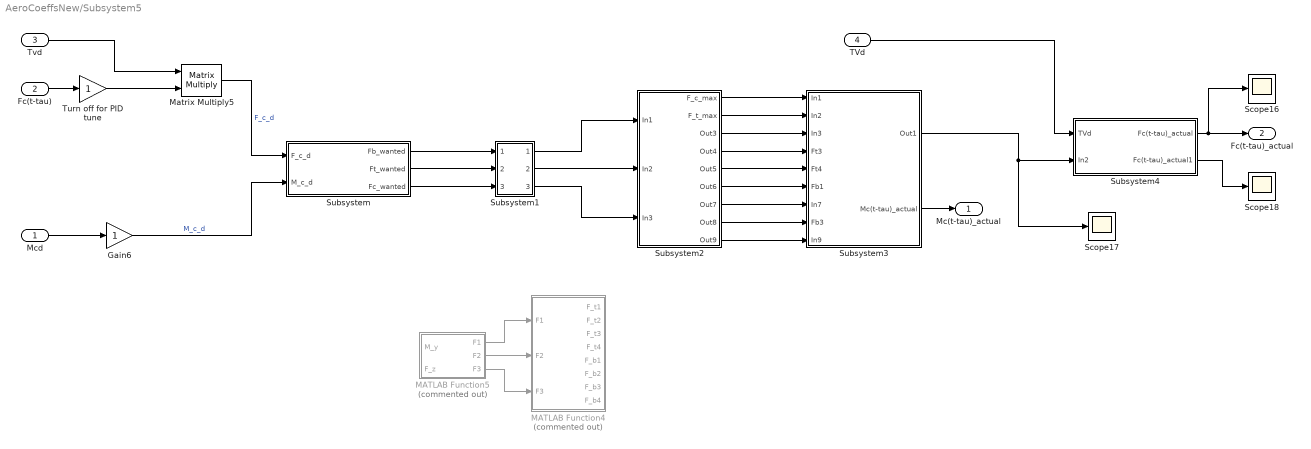
== system AeroCoeffsNew/Subsystem5 ==
  Mcd : Inport
  Fc(t-tau) : Inport  Port=2
  Tvd : Inport  Port=3
  TVd : Inport  Port=4
  Gain6 : Gain
  MATLAB Function4 : MATLAB Function  Commented=on  TreatAsAtomicUnit=on
  MATLAB Function5 : MATLAB Function  Commented=on  TreatAsAtomicUnit=on
  Matrix Multiply5 : Product  Multiplication=Matrix(*)
  Scope16 : Scope
  Scope17 : Scope
  Scope18 : Scope
  Subsystem : Subsystem
  Subsystem1 : Subsystem
  Subsystem2 : Subsystem
  Subsystem3 : Subsystem
  Subsystem4 : Subsystem
  Turn off for PID tune : Gain
  Mc(t-tau)_actual : Outport
  Fc(t-tau)_actual : Outport  Port=2
  wires:
  Mcd/1 -> Gain6/1
  Turn off for PID tune/1 -> Matrix Multiply5/2
  Tvd/1 -> Matrix Multiply5/1
  Fc(t-tau)/1 -> Turn off for PID tune/1
  MATLAB Function5/1(F1) -> MATLAB Function4/1(F1)
  MATLAB Function5/3(F3) -> MATLAB Function4/3(F3)
  MATLAB Function5/2(F2) -> MATLAB Function4/2(F2)
  Matrix Multiply5/1 -> Subsystem/1(F_c_d)  "F_c_d"
  Gain6/1 -> Subsystem/2(M_c_d)  "M_c_d"
  Subsystem/1(Fb_wanted) -> Subsystem1/1(In1)
  Subsystem/2(Ft_wanted) -> Subsystem1/2(In2)
  Subsystem/3(Fc_wanted) -> Subsystem1/3(In3)
  Subsystem1/1(Out1) -> Subsystem2/1(In1)
  Subsystem1/2(Out2) -> Subsystem2/2(In2)
  Subsystem1/3(Out3) -> Subsystem2/3(In3)
  Subsystem3/1(Out1) -> Scope17/1, Subsystem4/2(In2)
  Subsystem2/1(F_c_max) -> Subsystem3/1(In1)
  Subsystem2/2(F_t_max) -> Subsystem3/2(In2)
  Subsystem2/3(Out3) -> Subsystem3/3(In3)
  Subsystem2/4(Out4) -> Subsystem3/4(Ft3)
  Subsystem2/5(Out5) -> Subsystem3/5(Ft4)
  Subsystem2/6(Out6) -> Subsystem3/6(Fb1)
  Subsystem2/7(Out7) -> Subsystem3/7(In7)
  Subsystem2/8(Out8) -> Subsystem3/8(Fb3)
  Subsystem2/9(Out9) -> Subsystem3/9(In9)
  Subsystem3/2(Mc(t-tau)_actual) -> Mc(t-tau)_actual/1
  Subsystem4/1(Fc(t-tau)_actual) -> Scope16/1, Fc(t-tau)_actual/1
  TVd/1 -> Subsystem4/1(TVd)
  Subsystem4/2(Fc(t-tau)_actual1) -> Scope18/1

== system AeroCoeffsNew/Subsystem7 ==
  Constant2 : Constant  Value=r_trajectory
  Constant9 : Constant  Value=[0;0;0]
  r_trajectory : Outport
  "sigma, tau, upsilon" : Outport  Port=2
  wires:
  Constant2/1 -> r_trajectory/1
  Constant9/1 -> "sigma, tau, upsilon"/1  "sigma, tau, upsilon"

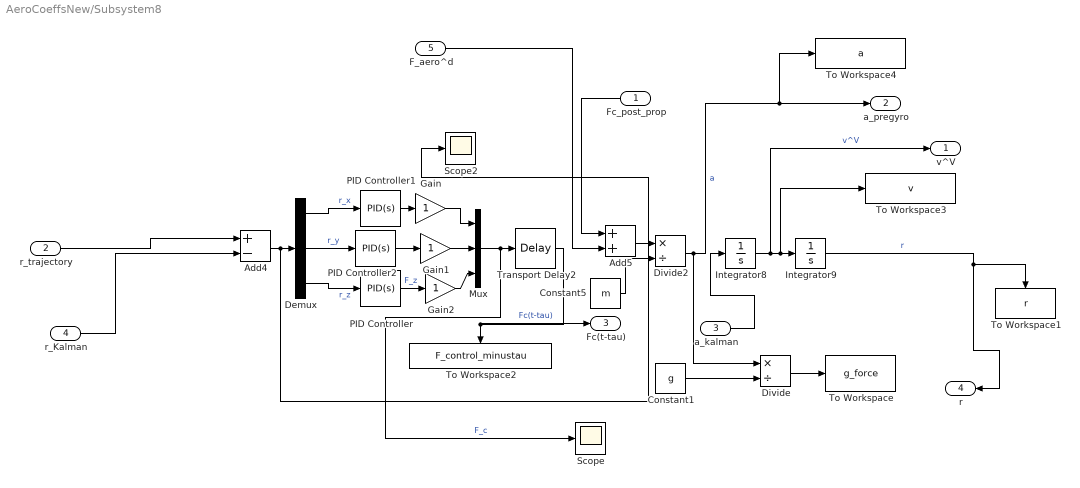
== system AeroCoeffsNew/Subsystem8 ==
  Fc_post_prop : Inport
  r_trajectory : Inport  Port=2
  a_kalman : Inport  Port=3
  r_Kalman : Inport  Port=4
  F_aero^d : Inport  Port=5
  Add4 : Sum  Inputs=+-
  Add5 : Sum
  Constant1 : Constant  Value=g
  Constant5 : Constant  Value=m
  Demux : Demux  Outputs=3
  Divide : Product  Inputs=*/
  Divide2 : Product  Inputs=*/
  Gain : Gain
  Gain1 : Gain
  Gain2 : Gain
  Integrator8 : Integrator  InitialCondition=v_0
  Integrator9 : Integrator  InitialCondition=r_0
  Mux : Mux  Inputs=3
  PID Controller : pid_lib/PID Controller  Controller=PID  Form=Parallel  TimeDomain=Continuous-time  UseExternalTs=off  SampleTime=-1  IntegratorMethod=Forward Euler  FilterMethod=Forward Euler  ControllerParametersSource=internal  P=160.734193661502  I=6.85755125615993  D=923.025793270617  UseFilter=on  N=10.4897155810233  TunerSelectOption=Transfer Function Based (PID Tuner App)  InitialConditionSource=internal  InitialConditionForIntegrator=0  InitialConditionForFilter=0  DifferentiatorICPrevScaledInput=0  ExternalReset=none  TrackingMode=off  Kt=1  LimitOutput=off  SatLimitsSource=internal  UpperSaturationLimit=inf  LowerSaturationLimit=-inf  LinearizeAsGain=on  AntiWindupMode=none  Kb=1  POutMin=[]  POutMax=[]  IOutMin=[]  IOutMax=[]  DOutMin=[]  DOutMax=[]  NOutMin=[]  NOutMax=[]  SumOutMin=[]  SumOutMax=[]  SaturationOutMin=[]  SaturationOutMax=[]  PParamMin=[]  PParamMax=[]  IParamMin=[]  IParamMax=[]  DParamMin=[]  DParamMax=[]  NParamMin=[]  NParamMax=[]  KbParamMin=[]  KbParamMax=[]  KtParamMin=[]  KtParamMax=[]  KbOutMin=[]  KbOutMax=[]  KtOutMin=[]  KtOutMax=[]  IntegratorOutMin=[]  IntegratorOutMax=[]  FilterOutMin=[]  FilterOutMax=[]  SumI1OutMin=[]  SumI1OutMax=[]  SumI2OutMin=[]  SumI2OutMax=[]  SumI3OutMin=[]  SumI3OutMax=[]  SumI4OutMin=[]  SumI4OutMax=[]  SumDOutMin=[]  SumDOutMax=[]  DifferentiatorOutMin=[]  DifferentiatorOutMax=[]  FilterDiffOutCoefMin=[]  FilterDiffOutCoefMax=[]  ReciprocalOutMin=[]  ReciprocalOutMax=[]  SumDenOutMin=[]  SumDenOutMax=[]  SumNumOutMin=[]  SumNumOutMax=[]  DivideOutMin=[]  DivideOutMax=[]  UdiffTsProdOutMin=[]  UdiffTsProdOutMax=[]  NTsProdOutMin=[]  NTsProdOutMax=[]  UintegralTsProdOutMin=[]  UintegralTsProdOutMax=[]  UngainTsProdOutMin=[]  UngainTsProdOutMax=[]  IntegratorContinuousStateAttributes=''  IntegratorStateMustResolveToSignalObject=off  IntegratorRTWStateStorageClass=Auto  FilterContinuousStateAttributes=''  FilterStateMustResolveToSignalObject=off  FilterRTWStateStorageClass=Auto  ParallelPVariant=InternalParameters  IdealPVariant=Disabled  IVariant=InternalParameters  DVariant=InternalParameters  IntegratorVariant=Continuous  SatVariant=Disabled  AWVariant=Passthrough  PCopyVariant=Disabled  TRVariant=Disabled  FdbkBlocksVariant=Forward  IdealPFdbkVariant=Disabled  SatFdbkVariant=Disabled  DerivativeFilterVariant=ContFilter  NVariant=InternalParameters  NCopyVariant=Disabled  FilterICVariant=InternalICsFilter  IntegratorICVariant=InternalICs  ExternalResetVariant=Disabled  TRSumVariant=Passthrough  SumFdbkVariant=Disabled  SumVariant=Sum_PID  TsampFilterVariant=InternalTs  TsampNgainVariant=Passthrough  TsampIntegralVariant=Passthrough  ExternalSaturationOutDataTypeStr=Inherit: Same as second input
  PID Controller1 : pid_lib/PID Controller  Controller=PID  Form=Parallel  TimeDomain=Continuous-time  UseExternalTs=off  SampleTime=-1  IntegratorMethod=Forward Euler  FilterMethod=Forward Euler  ControllerParametersSource=internal  P=160.734193661502  I=6.85755125615993  D=923.025793270617  UseFilter=on  N=10.4897155810233  TunerSelectOption=Transfer Function Based (PID Tuner App)  InitialConditionSource=internal  InitialConditionForIntegrator=0  InitialConditionForFilter=0  DifferentiatorICPrevScaledInput=0  ExternalReset=none  TrackingMode=off  Kt=1  LimitOutput=off  SatLimitsSource=internal  UpperSaturationLimit=inf  LowerSaturationLimit=-inf  LinearizeAsGain=on  AntiWindupMode=none  Kb=1  POutMin=[]  POutMax=[]  IOutMin=[]  IOutMax=[]  DOutMin=[]  DOutMax=[]  NOutMin=[]  NOutMax=[]  SumOutMin=[]  SumOutMax=[]  SaturationOutMin=[]  SaturationOutMax=[]  PParamMin=[]  PParamMax=[]  IParamMin=[]  IParamMax=[]  DParamMin=[]  DParamMax=[]  NParamMin=[]  NParamMax=[]  KbParamMin=[]  KbParamMax=[]  KtParamMin=[]  KtParamMax=[]  KbOutMin=[]  KbOutMax=[]  KtOutMin=[]  KtOutMax=[]  IntegratorOutMin=[]  IntegratorOutMax=[]  FilterOutMin=[]  FilterOutMax=[]  SumI1OutMin=[]  SumI1OutMax=[]  SumI2OutMin=[]  SumI2OutMax=[]  SumI3OutMin=[]  SumI3OutMax=[]  SumI4OutMin=[]  SumI4OutMax=[]  SumDOutMin=[]  SumDOutMax=[]  DifferentiatorOutMin=[]  DifferentiatorOutMax=[]  FilterDiffOutCoefMin=[]  FilterDiffOutCoefMax=[]  ReciprocalOutMin=[]  ReciprocalOutMax=[]  SumDenOutMin=[]  SumDenOutMax=[]  SumNumOutMin=[]  SumNumOutMax=[]  DivideOutMin=[]  DivideOutMax=[]  UdiffTsProdOutMin=[]  UdiffTsProdOutMax=[]  NTsProdOutMin=[]  NTsProdOutMax=[]  UintegralTsProdOutMin=[]  UintegralTsProdOutMax=[]  UngainTsProdOutMin=[]  UngainTsProdOutMax=[]  IntegratorContinuousStateAttributes=''  IntegratorStateMustResolveToSignalObject=off  IntegratorRTWStateStorageClass=Auto  FilterContinuousStateAttributes=''  FilterStateMustResolveToSignalObject=off  FilterRTWStateStorageClass=Auto  ParallelPVariant=InternalParameters  IdealPVariant=Disabled  IVariant=InternalParameters  DVariant=InternalParameters  IntegratorVariant=Continuous  SatVariant=Disabled  AWVariant=Passthrough  PCopyVariant=Disabled  TRVariant=Disabled  FdbkBlocksVariant=Forward  IdealPFdbkVariant=Disabled  SatFdbkVariant=Disabled  DerivativeFilterVariant=ContFilter  NVariant=InternalParameters  NCopyVariant=Disabled  FilterICVariant=InternalICsFilter  IntegratorICVariant=InternalICs  ExternalResetVariant=Disabled  TRSumVariant=Passthrough  SumFdbkVariant=Disabled  SumVariant=Sum_PID  TsampFilterVariant=InternalTs  TsampNgainVariant=Passthrough  TsampIntegralVariant=Passthrough  ExternalSaturationOutDataTypeStr=Inherit: Same as second input
  PID Controller2 : pid_lib/PID Controller  Controller=PID  Form=Parallel  TimeDomain=Continuous-time  UseExternalTs=off  SampleTime=-1  IntegratorMethod=Forward Euler  FilterMethod=Forward Euler  ControllerParametersSource=internal  P=160.734193661502*2  I=6.85755125615993  D=923.025793270617  UseFilter=on  N=10.4897155810233  TunerSelectOption=Transfer Function Based (PID Tuner App)  InitialConditionSource=internal  InitialConditionForIntegrator=0  InitialConditionForFilter=0  DifferentiatorICPrevScaledInput=0  ExternalReset=none  TrackingMode=off  Kt=1  LimitOutput=off  SatLimitsSource=internal  UpperSaturationLimit=inf  LowerSaturationLimit=-inf  LinearizeAsGain=on  AntiWindupMode=none  Kb=1  POutMin=[]  POutMax=[]  IOutMin=[]  IOutMax=[]  DOutMin=[]  DOutMax=[]  NOutMin=[]  NOutMax=[]  SumOutMin=[]  SumOutMax=[]  SaturationOutMin=[]  SaturationOutMax=[]  PParamMin=[]  PParamMax=[]  IParamMin=[]  IParamMax=[]  DParamMin=[]  DParamMax=[]  NParamMin=[]  NParamMax=[]  KbParamMin=[]  KbParamMax=[]  KtParamMin=[]  KtParamMax=[]  KbOutMin=[]  KbOutMax=[]  KtOutMin=[]  KtOutMax=[]  IntegratorOutMin=[]  IntegratorOutMax=[]  FilterOutMin=[]  FilterOutMax=[]  SumI1OutMin=[]  SumI1OutMax=[]  SumI2OutMin=[]  SumI2OutMax=[]  SumI3OutMin=[]  SumI3OutMax=[]  SumI4OutMin=[]  SumI4OutMax=[]  SumDOutMin=[]  SumDOutMax=[]  DifferentiatorOutMin=[]  DifferentiatorOutMax=[]  FilterDiffOutCoefMin=[]  FilterDiffOutCoefMax=[]  ReciprocalOutMin=[]  ReciprocalOutMax=[]  SumDenOutMin=[]  SumDenOutMax=[]  SumNumOutMin=[]  SumNumOutMax=[]  DivideOutMin=[]  DivideOutMax=[]  UdiffTsProdOutMin=[]  UdiffTsProdOutMax=[]  NTsProdOutMin=[]  NTsProdOutMax=[]  UintegralTsProdOutMin=[]  UintegralTsProdOutMax=[]  UngainTsProdOutMin=[]  UngainTsProdOutMax=[]  IntegratorContinuousStateAttributes=''  IntegratorStateMustResolveToSignalObject=off  IntegratorRTWStateStorageClass=Auto  FilterContinuousStateAttributes=''  FilterStateMustResolveToSignalObject=off  FilterRTWStateStorageClass=Auto  ParallelPVariant=InternalParameters  IdealPVariant=Disabled  IVariant=InternalParameters  DVariant=InternalParameters  IntegratorVariant=Continuous  SatVariant=Disabled  AWVariant=Passthrough  PCopyVariant=Disabled  TRVariant=Disabled  FdbkBlocksVariant=Forward  IdealPFdbkVariant=Disabled  SatFdbkVariant=Disabled  DerivativeFilterVariant=ContFilter  NVariant=InternalParameters  NCopyVariant=Disabled  FilterICVariant=InternalICsFilter  IntegratorICVariant=InternalICs  ExternalResetVariant=Disabled  TRSumVariant=Passthrough  SumFdbkVariant=Disabled  SumVariant=Sum_PID  TsampFilterVariant=InternalTs  TsampNgainVariant=Passthrough  TsampIntegralVariant=Passthrough  ExternalSaturationOutDataTypeStr=Inherit: Same as second input
  Scope : Scope
  Scope2 : Scope
  To Workspace : ToWorkspace  VariableName=g_force  SaveFormat=Timeseries  SampleTime=-1
      settings: Save2DSignal=2-D array (concatenate along first dimension)
  To Workspace1 : ToWorkspace  VariableName=r  SaveFormat=Timeseries  SampleTime=-1
  To Workspace2 : ToWorkspace  VariableName=F_control_minustau  SaveFormat=Timeseries  SampleTime=-1
  To Workspace3 : ToWorkspace  VariableName=v  SaveFormat=Timeseries  SampleTime=-1
  To Workspace4 : ToWorkspace  VariableName=a  SaveFormat=Timeseries  SampleTime=-1
  Transport Delay2 : TransportDelay  DelayTime=time_delay  TransDelayFeedthrough=on
  v^V : Outport
  a_pregyro : Outport  Port=2
  Fc(t-tau) : Outport  Port=3
  r : Outport  Port=4
  wires:
  Add5/1 -> Divide2/1
  PID Controller1/1 -> Gain/1
  a_kalman/1 -> Integrator8/1
  Gain/1 -> Mux/1
  Integrator8/1 -> v^V/1, To Workspace3/1, Integrator9/1  "v^V"
  Gain2/1 -> Mux/3
  F_aero^d/1 -> Add5/2
  r_trajectory/1 -> Add4/1
  PID Controller/1 -> Gain2/1  "F_z"
  Add4/1 -> Scope2/1, Demux/1
  Integrator9/1 -> r/1, To Workspace1/1  "r"
  Mux/1 -> Scope/1, Transport Delay2/1  "F_c"
  Gain1/1 -> Mux/2
  Constant5/1 -> Divide2/2
  Demux/2 -> PID Controller2/1  "r_y"
  PID Controller2/1 -> Gain1/1
  r_Kalman/1 -> Add4/2
  Demux/1 -> PID Controller1/1  "r_x"
  Demux/3 -> PID Controller/1  "r_z"
  Divide/1 -> To Workspace/1
  Constant1/1 -> Divide/2
  Transport Delay2/1 -> To Workspace2/1, Fc(t-tau)/1  "Fc(t-tau)"
  Divide2/1 -> To Workspace4/1, a_pregyro/1, Divide/1  "a"
  Fc_post_prop/1 -> Add5/1

== system AeroCoeffsNew/Subsystem9 ==
  a_sensed : Inport
  position : Inport  Port=2
  Fc(t-tau) : Inport  Port=3
  Add : Sum  Inputs=+-
  Add1 : Sum  Inputs=+-
  Add2 : Sum  Inputs=+-
  Add3 : Sum
  GPS Model : MATLAB Function  TreatAsAtomicUnit=on
  Gain : Gain  Gain=0
  Gain1 : Gain
  Subsystem6 : Subsystem
  To Workspace : ToWorkspace  VariableName=GPS_error  SaveFormat=Timeseries  SampleTime=-1
  To Workspace1 : ToWorkspace  VariableName=Kal_tot  SaveFormat=Timeseries  SampleTime=-1
  To Workspace2 : ToWorkspace  VariableName=Kal_GPS  SaveFormat=Timeseries  SampleTime=-1
  Transpose : Math  Operator=transpose  SaturateOnIntegerOverflow=on
  r_kalman : Outport
  wires:
  GPS Model/1(newposition) -> Transpose/1, Gain1/1, Add2/2, Subsystem6/3(gps error)  "gps error"
  Fc(t-tau)/1 -> Subsystem6/1(Fc(t-tau))
  Subsystem6/1(r_kalman) -> Add2/1, Add1/2, Gain/1
  position/1 -> Add/1, Add1/1, GPS Model/1(position)
  a_sensed/1 -> Subsystem6/2(a_sensed)
  Add/1 -> To Workspace/1
  Add1/1 -> To Workspace1/1
  Add2/1 -> To Workspace2/1
  Transpose/1 -> Add/2
  Gain/1 -> Add3/1
  Gain1/1 -> Add3/2
  Add3/1 -> r_kalman/1

== system AeroCoeffsNew/Wind gust1 ==
  Add : Sum  Inputs=+-
  Add1 : Sum  Inputs=+-
  Constant : Constant  Value=12.4
  Constant1 : Constant  Value=4.25
  Constant2 : Constant
  Constant3 : Constant  Value=0
  Constant4 : Constant  Value=0  VectorParams1D=off
  Mux : Mux  Inputs=3
  Product : Product
  Product1 : Product
  Sine Wave : Sin  Frequency=3*pi/T  SampleTime=0
  Sine Wave1 : Sin  Frequency=2*pi/T  Phase=pi/2  SampleTime=0
  V_tot : Outport
  wires:
  Constant/1 -> Add/1
  Constant1/1 -> Product/1
  Sine Wave/1 -> Product/2
  Constant2/1 -> Add1/1
  Sine Wave1/1 -> Add1/2
  Product/1 -> Product1/1
  Add1/1 -> Product1/2
  Product1/1 -> Add/2
  Add/1 -> Mux/2  "v_gust_y"
  Constant3/1 -> Mux/3  "v_gust_z"
  Constant4/1 -> Mux/1  "v_gust_x"
  Mux/1 -> V_tot/1

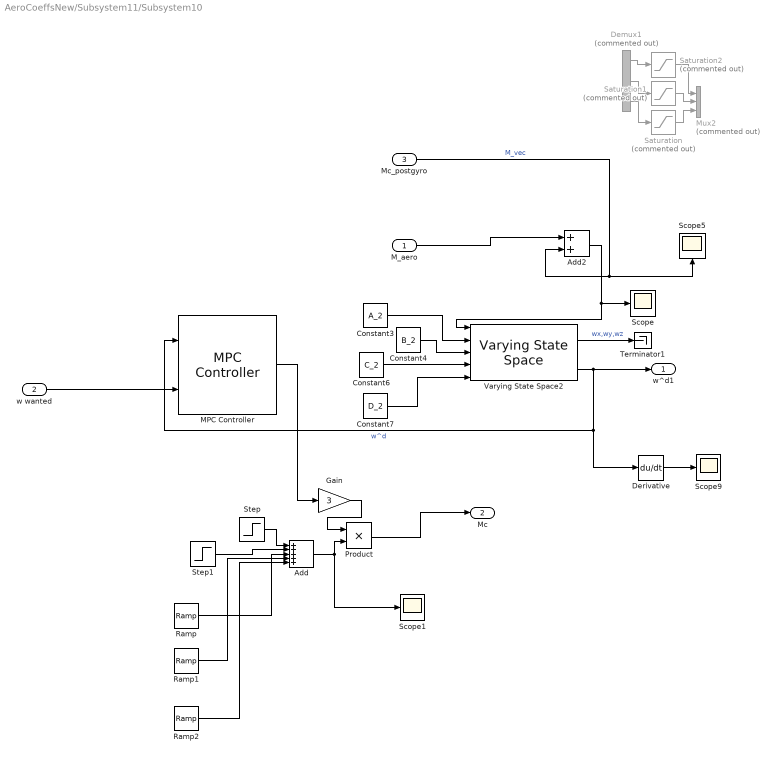
== system AeroCoeffsNew/Subsystem11/Subsystem10 ==
  M_aero : Inport
  w wanted : Inport  Port=2
  Mc_postgyro : Inport  Port=3
  Add : Sum  Inputs=+++++
  Add2 : Sum
  Constant3 : Constant  Value=A_2
  Constant4 : Constant  Value=B_2
  Constant6 : Constant  Value=C_2
  Constant7 : Constant  Value=D_2
  Demux1 : Demux  Commented=on  Outputs=3
  Derivative : Derivative
  Gain : Gain  Gain=3
  MPC Controller : mpclib/MPC Controller  SCDEnableBlockLinearizationSpecification=on  mpcobj=MPCDesignerSession.AppData.Controllers.MPC  is_multiple=0  enable_value=0  return_u0=off  updateMPCinCallerWorkspace=on  md_inport=off  mv_inport=off  uref_inport=off  return_cost=off  return_mvseq=off  return_qpstatus=off  return_xseq=off  return_state=off  return_ovseq=off  state_inport=off  umin_inport=off  umax_inport=off  ymin_inport=off  ymax_inport=off  cc_inport=off  ywt_inport=off  uwt_inport=off  duwt_inport=off  rhoeps_inport=off  pm_inport=off  MaximumP=10  HorizonChoice=FixedHorizon  n_ts=0.1  n_p=10  n_mv=3  n_md=0  n_ud=0  n_mo=3  n_uo=0  BlockDataType=double  SampleTimeInherited=off  switch_inport=off
  Mux2 : Mux  Commented=on  Inputs=3
  Product : Product
  Ramp : simulink/Sources/Ramp  slope=-0.1  start=time  InitialOutput=0
  Ramp1 : simulink/Sources/Ramp  slope=0.095  start=time+4  InitialOutput=0
  Ramp2 : simulink/Sources/Ramp  slope=0.005  start=time+4+15  InitialOutput=0
  Saturation : Saturate  Commented=on  UpperLimit=1000  LowerLimit=-1000
  Saturation1 : Saturate  Commented=on  UpperLimit=1000  LowerLimit=-1000
  Saturation2 : Saturate  Commented=on  UpperLimit=1000  LowerLimit=-1000
  Scope{,1,5,9} (4 alike) : Scope
  Step : Step  Time=0  SampleTime=0
  Step1 : Step  Time=time  After=-0.5  SampleTime=0
  Terminator1 : Terminator
  Varying State Space2 : cstblocks/Linear Parameter Varying/Varying State Space  x0=0  xNames=''  OutputX=on  OutputDX=off
  w^d1 : Outport
  Mc : Outport  Port=2
  wires:
  Constant6/1 -> Varying State Space2/4
  Varying State Space2/1 -> Terminator1/1  "wx,wy,wz"
  Constant4/1 -> Varying State Space2/3
  Add2/1 -> Scope/1, Varying State Space2/1
  Constant3/1 -> Varying State Space2/2
  Mc_postgyro/1 -> Scope5/1, Add2/2  "M_vec"
  Derivative/1 -> Scope9/1
  w wanted/1 -> MPC Controller/2
  Constant7/1 -> Varying State Space2/5
  Varying State Space2/2 -> w^d1/1, Derivative/1, MPC Controller/1  "w^d"
  M_aero/1 -> Add2/1
  Saturation/1 -> Mux2/3
  Demux1/2 -> Saturation1/1
  Saturation1/1 -> Mux2/2
  ? -> Demux1/1
  Demux1/3 -> Saturation/1
  Saturation2/1 -> Mux2/1
  Demux1/1 -> Saturation2/1
  Gain/1 -> Product/1
  MPC Controller/1 -> Gain/1
  Add/1 -> Scope1/1, Product/2
  Product/1 -> Mc/1
  Ramp/1 -> Add/3
  Step1/1 -> Add/2
  Step/1 -> Add/1
  Ramp1/1 -> Add/4
  Ramp2/1 -> Add/5
